simulink model "BLDC_FOC_SVPWM_Speed_and_Current_Control"  (R2013a)
settings: Solver=ode45  StartTime=0.0  StopTime=4  RelTol=1e-3
libraries: powerlib x7, simulink x5, simulink_extras x1, powerlib_meascontrol x1
settings Model: Creator=Sony  LastModifiedBy=Yooshaa

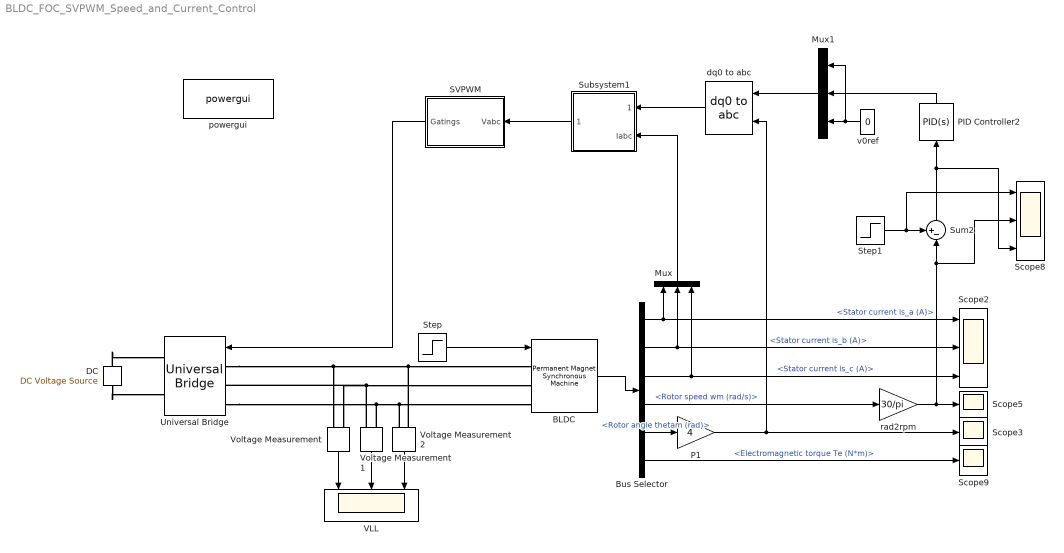
== system BLDC_FOC_SVPWM_Speed_and_Current_Control ==
  BLDC : powerlib/Machines/Permanent Magnet Synchronous Machine  NbPhases=3  FluxDistribution=Trapezoidal  RotorType=Round  MechanicalLoad=Torque Tm  PresetModel=No  ShowDetailedParameters=on  Resistance=0.01  Inductance=1e-4  dqInductances=[8.5e-3,8.5e-3]  La=0.000835  MachineConstant=Flux linkage established by magnets (V.s)  Flux=0.01  VoltageCst=8.3776  TorqueCst=0.08  Flat=120  Mechanical=[1e-3 1e-3 4 0]  PolePairs=4  InitialConditions=[0,0, 0,0]  InitialConditions5ph=[0 0 0 0 0 0]  TsPowergui=0  TsBlock=-1  RefAngle=Aligned with phase A axis (original Park)
  Bus Selector : BusSelector  OutputSignals=Stator current is_a (A),Stator current is_b (A),Stator current is_c (A),Rotor speed wm (rad/s),Rotor angle thetam (rad),Electromagnetic torque Te (N*m)
  DC : powerlib/Electrical Sources/DC Voltage Source  Amplitude=48  Measurements=None
  Mux : Mux  Inputs=3
  Mux1 : Mux  Inputs=3
  P1 : Gain  Gain=4
  PID Controller2 : simulink/Continuous/PID Controller  Controller=PID  TimeDomain=Continuous-time  SampleTime=1  IntegratorMethod=Forward Euler  FilterMethod=Forward Euler  Form=Parallel  P=0.1  I=1  D=0  N=100  InitialConditionSource=internal  InitialConditionForIntegrator=0  InitialConditionForFilter=0  ExternalReset=none  LimitOutput=on  UpperSaturationLimit=100  LowerSaturationLimit=-100  LinearizeAsGain=on  AntiWindupMode=none  Kb=1  TrackingMode=off  Kt=1  PParamMin=[]  PParamMax=[]  IParamMin=[]  IParamMax=[]  DParamMin=[]  DParamMax=[]  NParamMin=[]  NParamMax=[]  KbParamMin=[]  KbParamMax=[]  KtParamMin=[]  KtParamMax=[]  POutMin=[]  POutMax=[]  IOutMin=[]  IOutMax=[]  DOutMin=[]  DOutMax=[]  NOutMin=[]  NOutMax=[]  KbOutMin=[]  KbOutMax=[]  KtOutMin=[]  KtOutMax=[]  IntegratorOutMin=[]  IntegratorOutMax=[]  FilterOutMin=[]  FilterOutMax=[]  SumOutMin=[]  SumOutMax=[]  SumI1OutMin=[]  SumI1OutMax=[]  SumI2OutMin=[]  SumI2OutMax=[]  SumI3OutMin=[]  SumI3OutMax=[]  SumDOutMin=[]  SumDOutMax=[]  SaturationOutMin=[]  SaturationOutMax=[]  IntegratorContinuousStateAttributes=''  IntegratorStateMustResolveToSignalObject=off  IntegratorRTWStateStorageClass=Auto  FilterContinuousStateAttributes=''  FilterStateMustResolveToSignalObject=off  FilterRTWStateStorageClass=Auto
  SVPWM : Subsystem  mask{Fs=10000, Fsampling=10000, Vbase=48, Vdc=48}
  Scope2 : Scope  NumInputPorts=3
      settings: YMin=-250~-250~-250  YMax=300~300~300
  Scope3 : Scope
      settings: YMin=0  YMax=7000
  Scope5 : Scope
      settings: YMin=-7000  YMax=7000  SaveName=ScopeData5
  Scope8 : Scope  NumInputPorts=3
      settings: YMin=-5000~-5000~-500  YMax=5000~5000~500  SaveName=ScopeData10
  Scope9 : Scope
      settings: YMin=-10  YMax=10  SaveName=ScopeData11
  Step : Step  Time=2  After=0  SampleTime=0
  Step1 : Step  Time=2  Before=-4000  After=4000  SampleTime=0
  Subsystem1 : Subsystem
  Sum2 : Sum  Inputs=+-|
  Universal Bridge : powerlib/Power Electronics/Universal Bridge  Arms=3  SnubberResistance=5000  SnubberCapacitance=1e-6  Device=MOSFET / Diodes  Ron=1e-3  Lon=0  ForwardVoltages="[  0  0  ]"  ForwardVoltage=0  GTOparameters=[ 10e-6 , 20e-6 ]  IGBTparameters=[ 1e-6 , 2e-6 ]  Measurements=None  Measurements_2=None  converterType=Rectifier
  VLL : Scope  NumInputPorts=3
      settings: YMin=-100~-100~-100  YMax=100~100~100  SaveName=ScopeData3
  Voltage Measurement : powerlib/Measurements/Voltage Measurement  PhasorSimulation=off  OutputType=Complex  PSBequivalent=0
  Voltage Measurement1 : powerlib/Measurements/Voltage Measurement  PhasorSimulation=off  OutputType=Complex  PSBequivalent=0
  Voltage Measurement2 : powerlib/Measurements/Voltage Measurement  PhasorSimulation=off  OutputType=Complex  PSBequivalent=0
  dq0 to abc : powerlib_meascontrol/Transformations/dq0 to abc  Alignment=Aligned with phase A axis
  powergui : powerlib/powergui  Priority=2  SimulationMode=Discrete  SolverType=Backward Euler  SampleTime=1e-5  frequency=60  SPID=off  DisableSnubberDevices=off  DisableRonSwitches=off  DisableVfSwitches=off  SwTol=0  Interpol=off  DisplayEquations=off  frequencyindice=0  Pbase=100e6  ErrMax=1e-4  Iterations=50  UnitsV=kV  UnitsW=MW  FunctionMessages=off  echomessages=off  HookPort=off  EnableUseOfTLC=off  x0status=blocks  RestoreLinks=warning  ResistiveCurrentMeasurement=off  Frange=[0:2:500]  Ylog=off  Xlog=on  ShowGrid=off  save=off  variable=ZData  ZoomFFT=on  StartTime=0.0  cycles=1  DisplayStyle=1  fundamental=60  FreqAxis=off  MaxFrequency=1000  frequencyindicesteady=1  RmsSteady=1  display=off  Ts=0  methode=off
  rad2rpm : Gain  Gain=30/pi
  v0ref : Constant  Value=0
  wires:
  Bus Selector/1 -> Scope2/1, Mux/1  "<Stator current is_a (A)>"
  BLDC/1 -> Bus Selector/1
  Bus Selector/2 -> Scope2/2, Mux/2  "<Stator current is_b (A)>"
  Bus Selector/4 -> rad2rpm/1  "<Rotor speed wm (rad/s)>"
  Bus Selector/3 -> Scope2/3, Mux/3  "<Stator current is_c (A)>"
  Mux/1 -> Subsystem1/2(Iabc)
  Bus Selector/5 -> P1/1  "<Rotor angle thetam (rad)>"
  SVPWM/1(Gatings) -> Universal Bridge/1
  PID Controller2/1 -> Mux1/2
  Mux1/1 -> dq0 to abc/1
  v0ref/1 -> Mux1/1, Mux1/3
  P1/1 -> Scope3/1, dq0 to abc/2
  Voltage Measurement2/1 -> VLL/3
  Voltage Measurement1/1 -> VLL/2
  Voltage Measurement/1 -> VLL/1
  Step1/1 -> Scope8/1, Sum2/1
  Sum2/1 -> Scope8/3, PID Controller2/1
  dq0 to abc/1 -> Subsystem1/1(Iabc_ref)
  Subsystem1/1(Pulses) -> SVPWM/1(Vabc)
  rad2rpm/1 -> Scope5/1, Scope8/2, Sum2/2
  Step/1 -> BLDC/1
  Bus Selector/6 -> Scope9/1  "<Electromagnetic torque Te (N*m)>"
  connections:
  Universal Bridge/LConn1 -- Voltage Measurement2/LConn2 -- BLDC/LConn1 -- Voltage Measurement/LConn1
  Universal Bridge/LConn2 -- Voltage Measurement/LConn2 -- Voltage Measurement1/LConn1 -- BLDC/LConn2
  Universal Bridge/LConn3 -- Voltage Measurement1/LConn2 -- Voltage Measurement2/LConn1 -- BLDC/LConn3
  DC/RConn1 -- Universal Bridge/RConn1
  DC/LConn1 -- Universal Bridge/RConn2

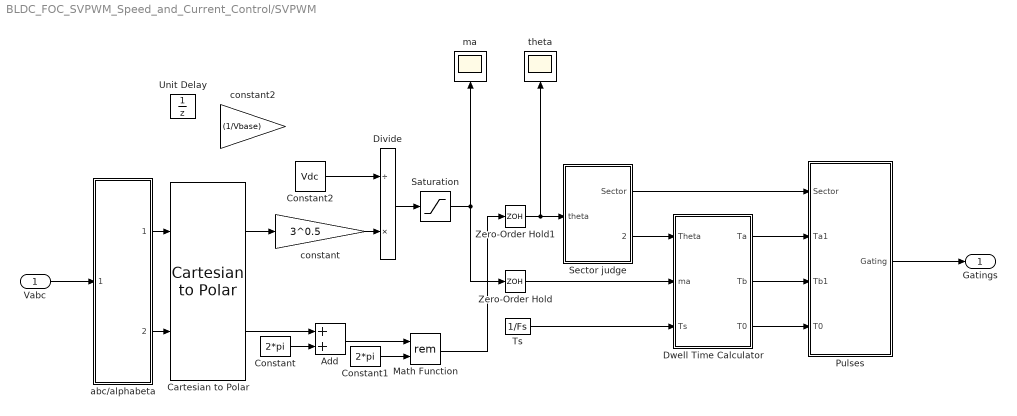
== system BLDC_FOC_SVPWM_Speed_and_Current_Control/SVPWM ==
  Vabc : Inport
  Add : Sum
  Cartesian to Polar : simulink_extras/Transformations/Cartesian to Polar
  Constant : Constant  Value=2*pi
  Constant1 : Constant  Value=2*pi
  Constant2 : Constant  Value=Vdc
  Divide : Product  Inputs=/*
  Dwell Time Calculator : Subsystem
  Math Function : Math  Operator=rem  SaturateOnIntegerOverflow=on
  Pulses : Subsystem
  Saturation : Saturate  UpperLimit=0.9  LowerLimit=0  SampleTime=1/Fsampling
  Sector judge : Subsystem
  Ts : Constant  Value=1/Fs
  Unit Delay : UnitDelay  InitialCondition=1220  SampleTime=1/Fsampling
  Zero-Order Hold : ZeroOrderHold  SampleTime=1/(2*Fs)
  Zero-Order Hold1 : ZeroOrderHold  SampleTime=1/(2*Fs)
  abc/alphabeta : Subsystem
  constant : Gain  Gain=3^0.5
  constant2 : Gain  Gain=(1/Vbase)
  ma : Scope
      settings: SaveName=ScopeData5
  theta : Scope
      settings: YMin=-3.5  YMax=3.5  SaveName=ScopeData6
  Gatings : Outport
  wires:
  Dwell Time Calculator/3(T0) -> Pulses/4(T0)
  constant/1 -> Divide/2
  Pulses/1(Gating) -> Gatings/1
  Cartesian to Polar/1 -> constant/1
  Divide/1 -> Saturation/1
  Ts/1 -> Dwell Time Calculator/3(Ts)
  Dwell Time Calculator/1(Ta) -> Pulses/2(Ta1)
  Dwell Time Calculator/2(Tb) -> Pulses/3(Tb1)
  Sector judge/2(Cal_theta) -> Dwell Time Calculator/1(Theta)
  Saturation/1 -> Zero-Order Hold/1, ma/1
  Zero-Order Hold/1 -> Dwell Time Calculator/2(ma)
  Constant2/1 -> Divide/1
  Zero-Order Hold1/1 -> Sector judge/1(theta), theta/1
  Sector judge/1(Sector) -> Pulses/1(Sector)
  abc/alphabeta/1(Valpha) -> Cartesian to Polar/1
  abc/alphabeta/2(Vbeta) -> Cartesian to Polar/2
  Cartesian to Polar/2 -> Add/1
  Math Function/1 -> Zero-Order Hold1/1
  Constant/1 -> Add/2
  Add/1 -> Math Function/1
  Constant1/1 -> Math Function/2
  Vabc/1 -> abc/alphabeta/1(Vabc)

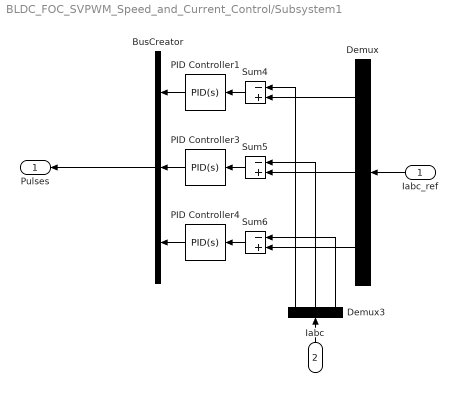
== system BLDC_FOC_SVPWM_Speed_and_Current_Control/Subsystem1 ==
  Iabc_ref : Inport
  Iabc : Inport  Port=2
  BusCreator : BusCreator  Inputs=3
  Demux : Demux  Outputs=3
  Demux3 : Demux  Outputs=3
  PID Controller1 : simulink/Continuous/PID Controller  Controller=PID  TimeDomain=Continuous-time  SampleTime=1  IntegratorMethod=Forward Euler  FilterMethod=Forward Euler  Form=Parallel  P=10  I=100  D=0  N=100  InitialConditionSource=internal  InitialConditionForIntegrator=0  InitialConditionForFilter=0  ExternalReset=none  LimitOutput=on  UpperSaturationLimit=48  LowerSaturationLimit=-48  LinearizeAsGain=on  AntiWindupMode=none  Kb=1  TrackingMode=off  Kt=1  PParamMin=[]  PParamMax=[]  IParamMin=[]  IParamMax=[]  DParamMin=[]  DParamMax=[]  NParamMin=[]  NParamMax=[]  KbParamMin=[]  KbParamMax=[]  KtParamMin=[]  KtParamMax=[]  POutMin=[]  POutMax=[]  IOutMin=[]  IOutMax=[]  DOutMin=[]  DOutMax=[]  NOutMin=[]  NOutMax=[]  KbOutMin=[]  KbOutMax=[]  KtOutMin=[]  KtOutMax=[]  IntegratorOutMin=[]  IntegratorOutMax=[]  FilterOutMin=[]  FilterOutMax=[]  SumOutMin=[]  SumOutMax=[]  SumI1OutMin=[]  SumI1OutMax=[]  SumI2OutMin=[]  SumI2OutMax=[]  SumI3OutMin=[]  SumI3OutMax=[]  SumDOutMin=[]  SumDOutMax=[]  SaturationOutMin=[]  SaturationOutMax=[]  IntegratorContinuousStateAttributes=''  IntegratorStateMustResolveToSignalObject=off  IntegratorRTWStateStorageClass=Auto  FilterContinuousStateAttributes=''  FilterStateMustResolveToSignalObject=off  FilterRTWStateStorageClass=Auto
  PID Controller3 : simulink/Continuous/PID Controller  Controller=PID  TimeDomain=Continuous-time  SampleTime=1  IntegratorMethod=Forward Euler  FilterMethod=Forward Euler  Form=Parallel  P=10  I=100  D=0  N=100  InitialConditionSource=internal  InitialConditionForIntegrator=0  InitialConditionForFilter=0  ExternalReset=none  LimitOutput=on  UpperSaturationLimit=48  LowerSaturationLimit=-48  LinearizeAsGain=on  AntiWindupMode=none  Kb=1  TrackingMode=off  Kt=1  PParamMin=[]  PParamMax=[]  IParamMin=[]  IParamMax=[]  DParamMin=[]  DParamMax=[]  NParamMin=[]  NParamMax=[]  KbParamMin=[]  KbParamMax=[]  KtParamMin=[]  KtParamMax=[]  POutMin=[]  POutMax=[]  IOutMin=[]  IOutMax=[]  DOutMin=[]  DOutMax=[]  NOutMin=[]  NOutMax=[]  KbOutMin=[]  KbOutMax=[]  KtOutMin=[]  KtOutMax=[]  IntegratorOutMin=[]  IntegratorOutMax=[]  FilterOutMin=[]  FilterOutMax=[]  SumOutMin=[]  SumOutMax=[]  SumI1OutMin=[]  SumI1OutMax=[]  SumI2OutMin=[]  SumI2OutMax=[]  SumI3OutMin=[]  SumI3OutMax=[]  SumDOutMin=[]  SumDOutMax=[]  SaturationOutMin=[]  SaturationOutMax=[]  IntegratorContinuousStateAttributes=''  IntegratorStateMustResolveToSignalObject=off  IntegratorRTWStateStorageClass=Auto  FilterContinuousStateAttributes=''  FilterStateMustResolveToSignalObject=off  FilterRTWStateStorageClass=Auto
  PID Controller4 : simulink/Continuous/PID Controller  Controller=PID  TimeDomain=Continuous-time  SampleTime=1  IntegratorMethod=Forward Euler  FilterMethod=Forward Euler  Form=Parallel  P=10  I=100  D=0  N=100  InitialConditionSource=internal  InitialConditionForIntegrator=0  InitialConditionForFilter=0  ExternalReset=none  LimitOutput=on  UpperSaturationLimit=48  LowerSaturationLimit=-48  LinearizeAsGain=on  AntiWindupMode=none  Kb=1  TrackingMode=off  Kt=1  PParamMin=[]  PParamMax=[]  IParamMin=[]  IParamMax=[]  DParamMin=[]  DParamMax=[]  NParamMin=[]  NParamMax=[]  KbParamMin=[]  KbParamMax=[]  KtParamMin=[]  KtParamMax=[]  POutMin=[]  POutMax=[]  IOutMin=[]  IOutMax=[]  DOutMin=[]  DOutMax=[]  NOutMin=[]  NOutMax=[]  KbOutMin=[]  KbOutMax=[]  KtOutMin=[]  KtOutMax=[]  IntegratorOutMin=[]  IntegratorOutMax=[]  FilterOutMin=[]  FilterOutMax=[]  SumOutMin=[]  SumOutMax=[]  SumI1OutMin=[]  SumI1OutMax=[]  SumI2OutMin=[]  SumI2OutMax=[]  SumI3OutMin=[]  SumI3OutMax=[]  SumDOutMin=[]  SumDOutMax=[]  SaturationOutMin=[]  SaturationOutMax=[]  IntegratorContinuousStateAttributes=''  IntegratorStateMustResolveToSignalObject=off  IntegratorRTWStateStorageClass=Auto  FilterContinuousStateAttributes=''  FilterStateMustResolveToSignalObject=off  FilterRTWStateStorageClass=Auto
  Sum4 : Sum  Inputs=-+  SaturateOnIntegerOverflow=on  InputSameDT=on  OutDataTypeStr=Inherit: Same as first input
  Sum5 : Sum  Inputs=-+  SaturateOnIntegerOverflow=on  InputSameDT=on  OutDataTypeStr=Inherit: Same as first input
  Sum6 : Sum  Inputs=-+  SaturateOnIntegerOverflow=on  InputSameDT=on  OutDataTypeStr=Inherit: Same as first input
  Pulses : Outport
  wires:
  Iabc/1 -> Demux3/1
  Demux/2 -> Sum5/2
  Demux/1 -> Sum4/2
  Demux3/2 -> Sum5/1
  Demux3/1 -> Sum4/1
  Demux3/3 -> Sum6/1
  Demux/3 -> Sum6/2
  Iabc_ref/1 -> Demux/1
  Sum4/1 -> PID Controller1/1
  Sum5/1 -> PID Controller3/1
  Sum6/1 -> PID Controller4/1
  BusCreator/1 -> Pulses/1
  PID Controller1/1 -> BusCreator/1
  PID Controller3/1 -> BusCreator/2
  PID Controller4/1 -> BusCreator/3

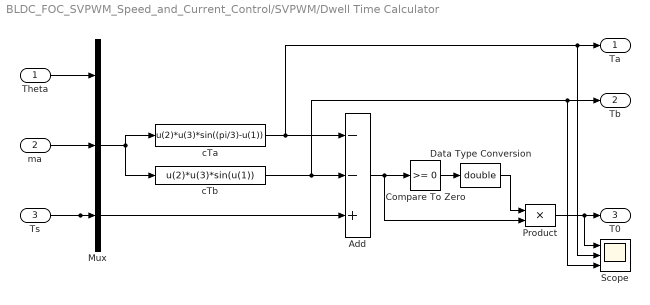
== system BLDC_FOC_SVPWM_Speed_and_Current_Control/SVPWM/Dwell Time Calculator ==
  Theta : Inport
  ma : Inport  Port=2
  Ts : Inport  Port=3
  Add : Sum  Inputs=--+
  Compare To Zero : simulink/Logic and Bit Operations/Compare To Zero  relop=>=  OutDataTypeStr=boolean
  Data Type Conversion : DataTypeConversion  OutDataTypeStr=double
  Mux : Mux  Inputs=3
  Product : Product  RndMeth=Zero
  Scope : Scope  NumInputPorts=3
      settings: YMin=-5~-5~-5  YMax=5~5~5  SaveName=ScopeData12
  cTa : Fcn  Expr=u(2)*u(3)*sin((pi/3)-u(1))
  cTb : Fcn  Expr=u(2)*u(3)*sin(u(1))
  Ta : Outport
  Tb : Outport  Port=2
  T0 : Outport  Port=3
  wires:
  Product/1 -> Scope/1, T0/1
  Theta/1 -> Mux/1
  ma/1 -> Mux/2
  Ts/1 -> Add/3, Mux/3
  Mux/1 -> cTb/1, cTa/1
  Add/1 -> Product/2, Compare To Zero/1
  Data Type Conversion/1 -> Product/1
  Compare To Zero/1 -> Data Type Conversion/1
  cTa/1 -> Scope/2, Ta/1, Add/1
  cTb/1 -> Scope/3, Tb/1, Add/2

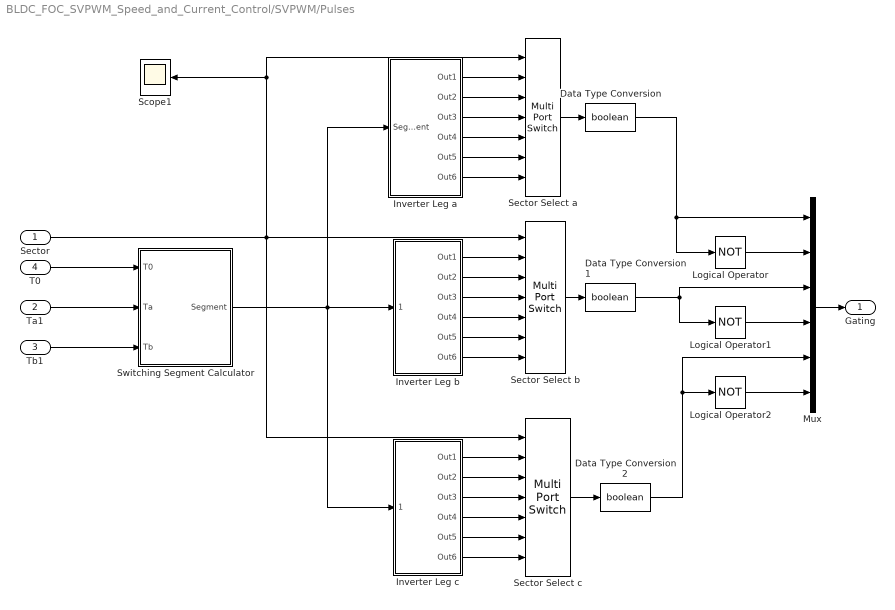
== system BLDC_FOC_SVPWM_Speed_and_Current_Control/SVPWM/Pulses ==
  Sector : Inport
  Ta1 : Inport  Port=2
  Tb1 : Inport  Port=3
  T0 : Inport  Port=4
  Data Type Conversion : DataTypeConversion  OutDataTypeStr=boolean  SaturateOnIntegerOverflow=on  RndMeth=Zero
  Data Type Conversion1 : DataTypeConversion  OutDataTypeStr=boolean  SaturateOnIntegerOverflow=on  RndMeth=Zero
  Data Type Conversion2 : DataTypeConversion  OutDataTypeStr=boolean  SaturateOnIntegerOverflow=on  RndMeth=Zero
  Inverter Leg a : Subsystem
  Inverter Leg b : Subsystem
  Inverter Leg c : Subsystem
  Logical Operator : Logic  Operator=NOT  AllPortsSameDT=off
  Logical Operator1 : Logic  Operator=NOT  AllPortsSameDT=off
  Logical Operator2 : Logic  Operator=NOT  AllPortsSameDT=off
  Mux : Mux  Inputs=6
  Scope1 : Scope
      settings: SaveName=ScopeData2
  Sector Select a : MultiPortSwitch  Inputs=6
  Sector Select b : MultiPortSwitch  Inputs=6
  Sector Select c : MultiPortSwitch  Inputs=6
  Switching Segment Calculator : Subsystem
  Gating : Outport
  wires:
  Sector/1 -> Sector Select a/1, Scope1/1, Sector Select b/1, Sector Select c/1
  Data Type Conversion/1 -> Logical Operator/1, Mux/1
  Data Type Conversion1/1 -> Mux/3, Logical Operator1/1
  Data Type Conversion2/1 -> Logical Operator2/1, Mux/5
  Mux/1 -> Gating/1
  Logical Operator/1 -> Mux/2
  Logical Operator1/1 -> Mux/4
  Logical Operator2/1 -> Mux/6
  Switching Segment Calculator/1(Segment) -> Inverter Leg c/1(Segment), Inverter Leg a/1(Segment), Inverter Leg b/1(Segment)
  T0/1 -> Switching Segment Calculator/1(T0)
  Ta1/1 -> Switching Segment Calculator/2(Ta)
  Tb1/1 -> Switching Segment Calculator/3(Tb)
  Inverter Leg a/1(Out1) -> Sector Select a/2
  Inverter Leg a/2(Out2) -> Sector Select a/3
  Inverter Leg a/3(Out3) -> Sector Select a/4
  Inverter Leg a/4(Out4) -> Sector Select a/5
  Inverter Leg a/5(Out5) -> Sector Select a/6
  Inverter Leg a/6(Out6) -> Sector Select a/7
  Inverter Leg b/1(Out1) -> Sector Select b/2
  Inverter Leg b/2(Out2) -> Sector Select b/3
  Inverter Leg b/3(Out3) -> Sector Select b/4
  Inverter Leg b/4(Out4) -> Sector Select b/5
  Inverter Leg b/5(Out5) -> Sector Select b/6
  Inverter Leg b/6(Out6) -> Sector Select b/7
  Inverter Leg c/1(Out1) -> Sector Select c/2
  Inverter Leg c/2(Out2) -> Sector Select c/3
  Inverter Leg c/3(Out3) -> Sector Select c/4
  Inverter Leg c/4(Out4) -> Sector Select c/5
  Inverter Leg c/5(Out5) -> Sector Select c/6
  Inverter Leg c/6(Out6) -> Sector Select c/7
  Sector Select a/1 -> Data Type Conversion/1
  Sector Select b/1 -> Data Type Conversion1/1
  Sector Select c/1 -> Data Type Conversion2/1

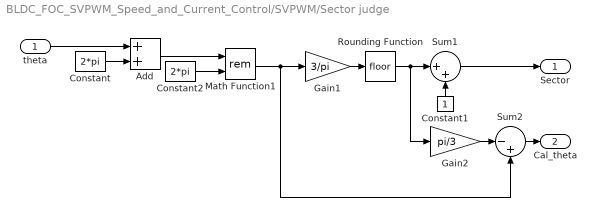
== system BLDC_FOC_SVPWM_Speed_and_Current_Control/SVPWM/Sector judge ==
  theta : Inport
  Add : Sum
  Constant : Constant  Value=2*pi
  Constant1 : Constant  OutDataTypeStr=boolean
  Constant2 : Constant  Value=2*pi
  Gain1 : Gain  Gain=3/pi
  Gain2 : Gain  Gain=pi/3
  Math Function1 : Math  Operator=rem  SaturateOnIntegerOverflow=on
  Rounding Function : Rounding
  Sum1 : Sum  Inputs=|++  SaturateOnIntegerOverflow=on
  Sum2 : Sum  Inputs=|-+
  Sector : Outport
  Cal_theta : Outport  Port=2
  wires:
  Gain1/1 -> Rounding Function/1
  Rounding Function/1 -> Gain2/1, Sum1/1
  Sum1/1 -> Sector/1
  Constant1/1 -> Sum1/2
  Gain2/1 -> Sum2/1
  Sum2/1 -> Cal_theta/1
  theta/1 -> Add/1
  Math Function1/1 -> Sum2/2, Gain1/1
  Constant/1 -> Add/2
  Add/1 -> Math Function1/1
  Constant2/1 -> Math Function1/2

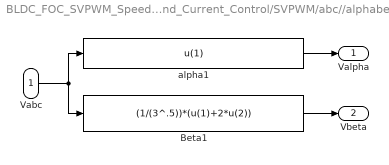
== system BLDC_FOC_SVPWM_Speed_and_Current_Control/SVPWM/abc//alphabeta ==
  Vabc : Inport
  Beta1 : Fcn  Expr=(1/(3^.5))*(u(1)+2*u(2))
  alpha1 : Fcn  Expr=u(1)
  Valpha : Outport
  Vbeta : Outport  Port=2
  wires:
  Vabc/1 -> Beta1/1, alpha1/1
  alpha1/1 -> Valpha/1
  Beta1/1 -> Vbeta/1

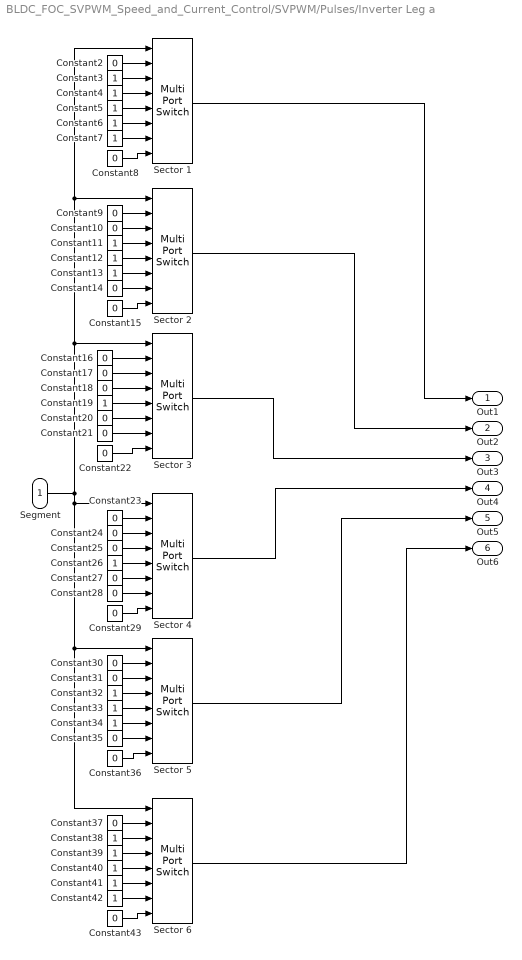
== system BLDC_FOC_SVPWM_Speed_and_Current_Control/SVPWM/Pulses/Inverter Leg a ==
  Segment : Inport
  Constant{2,8..10,14..18,20..25,27..31,35..37,43} (24 alike) : Constant  Value=0
  Constant{3..7,11..13,19,26,32..34,38..42} (18 alike) : Constant
  Sector {1..6} (6 alike) : MultiPortSwitch  Inputs=7
  Out1 : Outport
  Out2 : Outport  Port=2
  Out3 : Outport  Port=3
  Out4 : Outport  Port=4
  Out5 : Outport  Port=5
  Out6 : Outport  Port=6
  wires:
  Segment/1 -> Sector 6/1, Sector 5/1, Sector 4/1, Sector 2/1, Sector 1/1, Sector 3/1
  Sector 3/1 -> Out3/1
  Constant2/1 -> Sector 1/2
  Constant7/1 -> Sector 1/7
  Sector 1/1 -> Out1/1
  Constant3/1 -> Sector 1/3
  Constant6/1 -> Sector 1/6
  Constant10/1 -> Sector 2/3
  Sector 6/1 -> Out6/1
  Sector 2/1 -> Out2/1
  Constant5/1 -> Sector 1/5
  Constant9/1 -> Sector 2/2
  Constant4/1 -> Sector 1/4
  Constant8/1 -> Sector 1/8
  Sector 4/1 -> Out4/1
  Sector 5/1 -> Out5/1
  Constant42/1 -> Sector 6/7
  Constant43/1 -> Sector 6/8
  Constant40/1 -> Sector 6/5
  Constant37/1 -> Sector 6/2
  Constant41/1 -> Sector 6/6
  Constant39/1 -> Sector 6/4
  Constant17/1 -> Sector 3/3
  Constant30/1 -> Sector 5/2
  Constant38/1 -> Sector 6/3
  Constant29/1 -> Sector 4/8
  Constant28/1 -> Sector 4/7
  Constant31/1 -> Sector 5/3
  Constant25/1 -> Sector 4/4
  Constant20/1 -> Sector 3/6
  Constant26/1 -> Sector 4/5
  Constant32/1 -> Sector 5/4
  Constant33/1 -> Sector 5/5
  Constant36/1 -> Sector 5/8
  Constant18/1 -> Sector 3/4
  Constant14/1 -> Sector 2/7
  Constant13/1 -> Sector 2/6
  Constant34/1 -> Sector 5/6
  Constant24/1 -> Sector 4/3
  Constant11/1 -> Sector 2/4
  Constant16/1 -> Sector 3/2
  Constant21/1 -> Sector 3/7
  Constant12/1 -> Sector 2/5
  Constant19/1 -> Sector 3/5
  Constant35/1 -> Sector 5/7
  Constant22/1 -> Sector 3/8
  Constant23/1 -> Sector 4/2
  Constant15/1 -> Sector 2/8
  Constant27/1 -> Sector 4/6

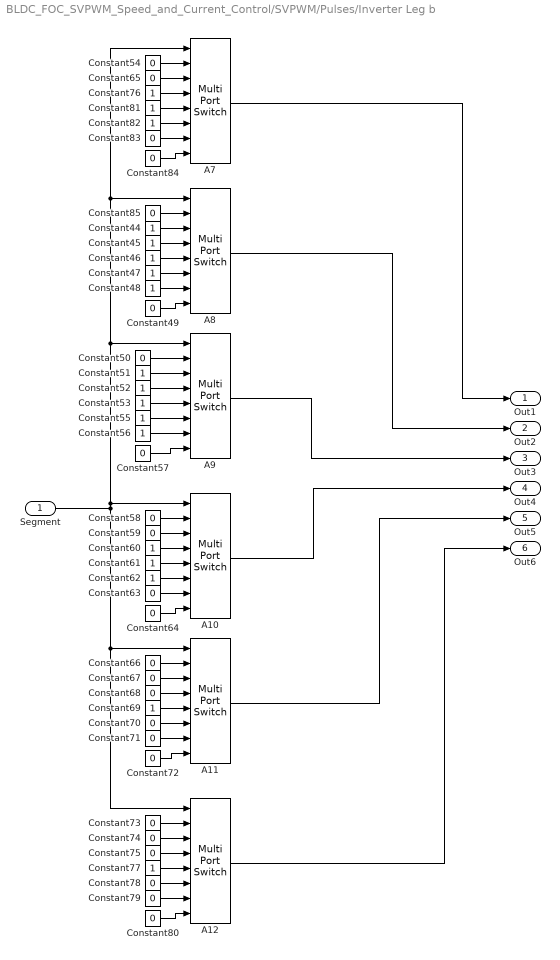
== system BLDC_FOC_SVPWM_Speed_and_Current_Control/SVPWM/Pulses/Inverter Leg b ==
  Segment : Inport
  A{7..12} (6 alike) : MultiPortSwitch  Inputs=7
  Constant{44..48,51..53,55..56,60..62,69,76..77,81..82} (18 alike) : Constant
  Constant{49..50,54,57..59,63..68,70..75,78..80,83..85} (24 alike) : Constant  Value=0
  Out1 : Outport
  Out2 : Outport  Port=2
  Out3 : Outport  Port=3
  Out4 : Outport  Port=4
  Out5 : Outport  Port=5
  Out6 : Outport  Port=6
  wires:
  Segment/1 -> A7/1, A8/1, A9/1, A10/1, A12/1, A11/1
  Constant80/1 -> A12/8
  Constant71/1 -> A11/7
  Constant69/1 -> A11/5
  Constant70/1 -> A11/6
  Constant72/1 -> A11/8
  Constant73/1 -> A12/2
  Constant75/1 -> A12/4
  Constant77/1 -> A12/5
  Constant79/1 -> A12/7
  Constant74/1 -> A12/3
  Constant68/1 -> A11/4
  Constant78/1 -> A12/6
  Constant55/1 -> A9/6
  Constant61/1 -> A10/5
  Constant47/1 -> A8/6
  Constant53/1 -> A9/5
  Constant45/1 -> A8/4
  Constant85/1 -> A8/2
  Constant49/1 -> A8/8
  Constant52/1 -> A9/4
  Constant56/1 -> A9/7
  Constant51/1 -> A9/3
  Constant57/1 -> A9/8
  Constant44/1 -> A8/3
  Constant46/1 -> A8/5
  Constant50/1 -> A9/2
  Constant48/1 -> A8/7
  Constant60/1 -> A10/4
  Constant62/1 -> A10/6
  Constant63/1 -> A10/7
  Constant64/1 -> A10/8
  Constant67/1 -> A11/3
  Constant66/1 -> A11/2
  Constant84/1 -> A7/8
  Constant59/1 -> A10/3
  Constant58/1 -> A10/2
  A9/1 -> Out3/1
  A8/1 -> Out2/1
  Constant65/1 -> A7/3
  A12/1 -> Out6/1
  A11/1 -> Out5/1
  A7/1 -> Out1/1
  Constant54/1 -> A7/2
  Constant76/1 -> A7/4
  A10/1 -> Out4/1
  Constant81/1 -> A7/5
  Constant82/1 -> A7/6
  Constant83/1 -> A7/7

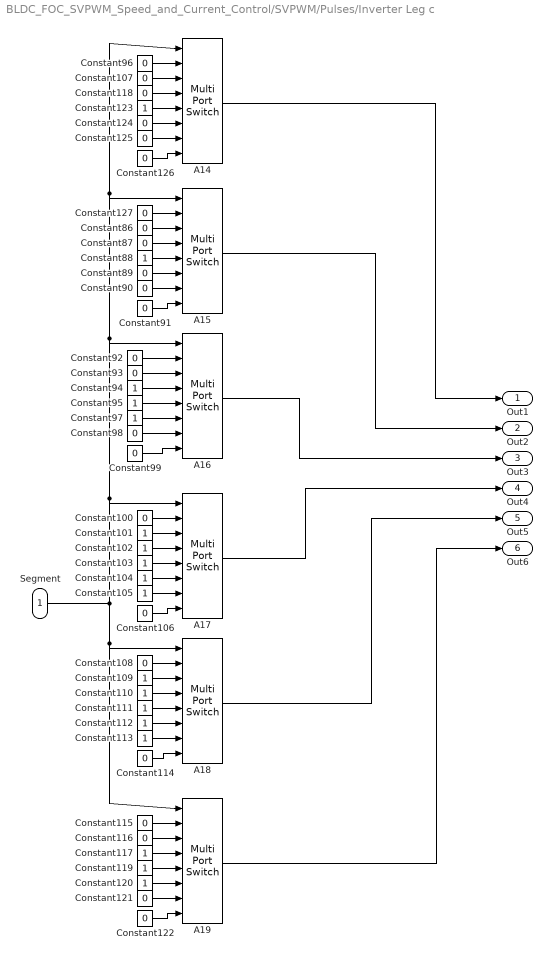
== system BLDC_FOC_SVPWM_Speed_and_Current_Control/SVPWM/Pulses/Inverter Leg c ==
  Segment : Inport
  A{14..19} (6 alike) : MultiPortSwitch  Inputs=7
  Constant{86..87,89..93,96,98..100,106..108,114..116,118,121..122,124..127} (24 alike) : Constant  Value=0
  Constant{88,94..95,97,101..105,109..113,117,119..120,123} (18 alike) : Constant
  Out1 : Outport
  Out2 : Outport  Port=2
  Out3 : Outport  Port=3
  Out4 : Outport  Port=4
  Out5 : Outport  Port=5
  Out6 : Outport  Port=6
  wires:
  Constant86/1 -> A15/3
  Constant103/1 -> A17/5
  Constant88/1 -> A15/5
  Constant101/1 -> A17/3
  Constant127/1 -> A15/2
  Constant102/1 -> A17/4
  Constant104/1 -> A17/6
  Constant100/1 -> A17/2
  Constant97/1 -> A16/6
  Constant94/1 -> A16/4
  Constant99/1 -> A16/8
  Constant105/1 -> A17/7
  Constant110/1 -> A18/4
  Constant109/1 -> A18/3
  Constant89/1 -> A15/6
  Constant113/1 -> A18/7
  Constant114/1 -> A18/8
  Constant87/1 -> A15/4
  Constant98/1 -> A16/7
  Constant91/1 -> A15/8
  Constant108/1 -> A18/2
  Constant92/1 -> A16/2
  Constant116/1 -> A19/3
  Constant111/1 -> A18/5
  Constant115/1 -> A19/2
  Constant117/1 -> A19/4
  Constant119/1 -> A19/5
  Constant112/1 -> A18/6
  Constant93/1 -> A16/3
  Constant95/1 -> A16/5
  Constant90/1 -> A15/7
  Constant106/1 -> A17/8
  Constant122/1 -> A19/8
  Constant121/1 -> A19/7
  Constant120/1 -> A19/6
  Segment/1 -> A15/1, A14/1, A16/1, A17/1, A19/1, A18/1
  Constant126/1 -> A14/8
  A16/1 -> Out3/1
  A17/1 -> Out4/1
  Constant96/1 -> A14/2
  Constant118/1 -> A14/4
  A18/1 -> Out5/1
  Constant107/1 -> A14/3
  A19/1 -> Out6/1
  Constant123/1 -> A14/5
  A15/1 -> Out2/1
  Constant124/1 -> A14/6
  A14/1 -> Out1/1
  Constant125/1 -> A14/7

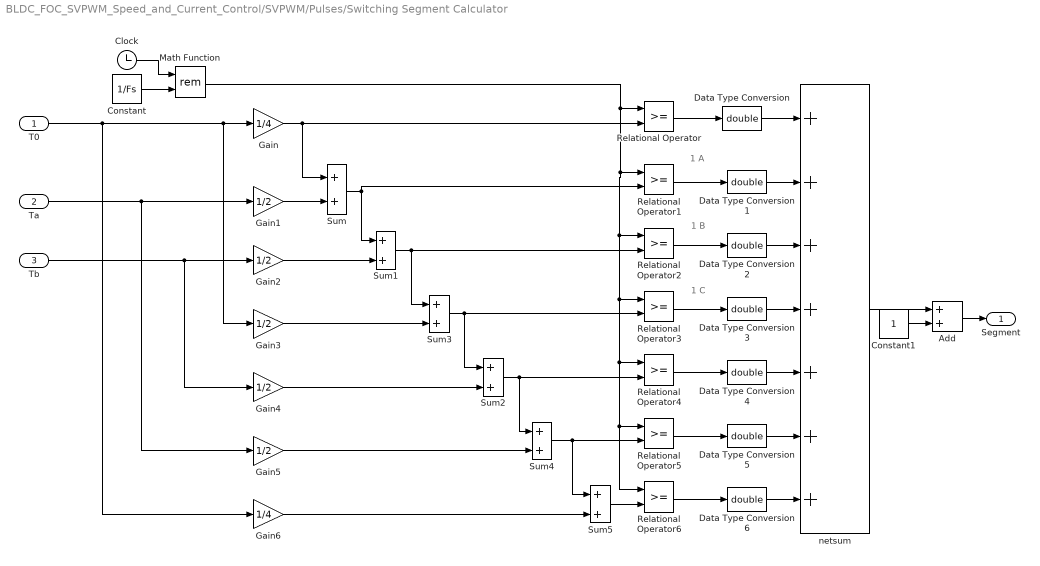
== system BLDC_FOC_SVPWM_Speed_and_Current_Control/SVPWM/Pulses/Switching Segment Calculator ==
  note: 1 A
  note: 1 B
  note: 1 C
  T0 : Inport
  Ta : Inport  Port=2
  Tb : Inport  Port=3
  Add : Sum
  Clock : Clock
  Constant : Constant  Value=1/Fs
  Constant1 : Constant
  Data Type Conversion{,1..6} (7 alike) : DataTypeConversion  OutDataTypeStr=double
  Gain : Gain  Gain=1/4
  Gain{1..5} (5 alike) : Gain  Gain=1/2
  Gain6 : Gain  Gain=1/4
  Math Function : Math  Operator=rem  SaturateOnIntegerOverflow=on
  Relational Operator{,1..6} (7 alike) : RelationalOperator  OutDataTypeStr=boolean
  Sum{,1..5} (6 alike) : Sum
  netsum : Sum  Inputs=7  SaturateOnIntegerOverflow=on  InputSameDT=on  OutDataTypeStr=Inherit: Same as first input
  Segment : Outport
  wires:
  Ta/1 -> Gain5/1, Gain1/1
  Gain2/1 -> Sum1/2
  Sum4/1 -> Sum5/1, Relational Operator5/2
  Math Function/1 -> Relational Operator6/1, Relational Operator5/1, Relational Operator4/1, Relational Operator3/1, Relational Operator2/1, Relational Operator1/1, Relational Operator/1
  Gain4/1 -> Sum2/2
  Gain5/1 -> Sum4/2
  Relational Operator/1 -> Data Type Conversion/1
  Relational Operator1/1 -> Data Type Conversion1/1
  Relational Operator2/1 -> Data Type Conversion2/1
  Sum3/1 -> Sum2/1, Relational Operator3/2
  Constant/1 -> Math Function/2
  Relational Operator3/1 -> Data Type Conversion3/1
  Gain3/1 -> Sum3/2
  Sum5/1 -> Relational Operator6/2
  Sum1/1 -> Sum3/1, Relational Operator2/2
  Gain6/1 -> Sum5/2
  Clock/1 -> Math Function/1
  Tb/1 -> Gain4/1, Gain2/1
  Sum/1 -> Sum1/1, Relational Operator1/2
  Gain/1 -> Sum/1, Relational Operator/2
  Gain1/1 -> Sum/2
  Sum2/1 -> Sum4/1, Relational Operator4/2
  Data Type Conversion3/1 -> netsum/4
  netsum/1 -> Add/1
  Data Type Conversion2/1 -> netsum/3
  Constant1/1 -> Add/2
  Data Type Conversion1/1 -> netsum/2
  Relational Operator4/1 -> Data Type Conversion4/1
  Data Type Conversion4/1 -> netsum/5
  Data Type Conversion6/1 -> netsum/7
  Data Type Conversion/1 -> netsum/1
  Relational Operator6/1 -> Data Type Conversion6/1
  Data Type Conversion5/1 -> netsum/6
  Relational Operator5/1 -> Data Type Conversion5/1
  Add/1 -> Segment/1
  T0/1 -> Gain6/1, Gain3/1, Gain/1
